simulink model "lotka_volterra"  (R2023a)
settings: Solver=VariableStepAuto  StartTime=0.0  StopTime=100  RelTol=1e-3
settings Model: Creator=vanes  LastModifiedBy=vanes
settings DataIOCC: ReturnWorkspaceOutputs=off  TimeSaveName=t

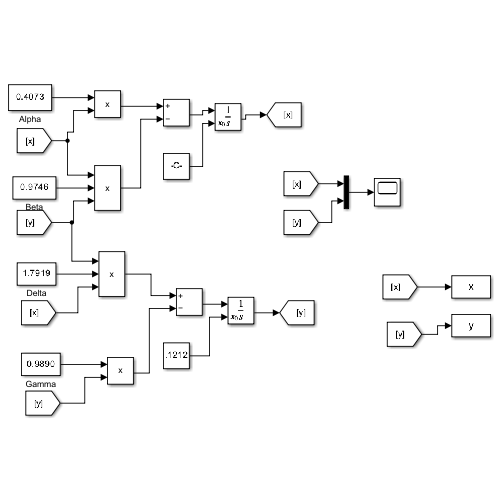
[thumbnail: Simulink's stored preview of the top-level diagram]
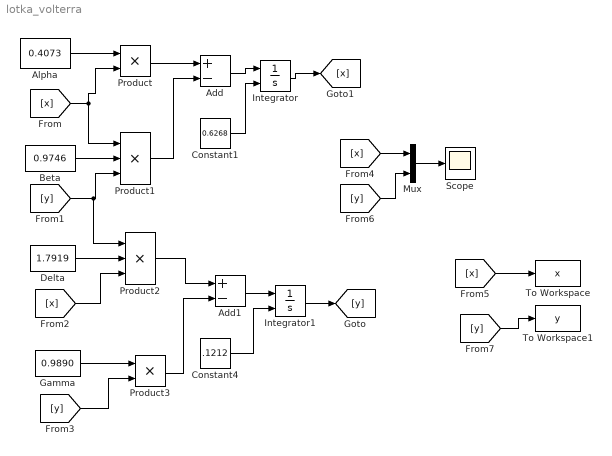
== system lotka_volterra ==
  Add : Sum  Inputs=+-
  Add1 : Sum  Inputs=+-
  Alpha : Constant  Value=0.4073
  Beta : Constant  Value=0.9746
  Constant1 : Constant  Value=0.6268
  Constant4 : Constant  Value=.1212
  Delta : Constant  Value=1.7919
  Gamma : Constant  Value=0.9890
  Integrator : Integrator  InitialConditionSource=external
  Integrator1 : Integrator  InitialConditionSource=external
  Mux : Mux  Inputs=2
  Product : Product
  Product1 : Product  Inputs=3
  Product2 : Product  Inputs=3
  Product3 : Product
  Scope : Scope
  To Workspace : ToWorkspace  VariableName=x  SampleTime=-1
  To Workspace1 : ToWorkspace  VariableName=y  SampleTime=-1
  wires:
  Alpha/1 -> Product/1
  [x] -> Product/2, Product1/1
  Beta/1 -> Product1/2
  [y] -> Product2/1, Product1/3
  Delta/1 -> Product2/2
  Product/1 -> Add/1
  Product1/1 -> Add/2
  Add/1 -> Integrator/1
  Integrator/1 -> [x]
  [x] -> Product2/3
  Gamma/1 -> Product3/1
  [y] -> Product3/2
  Constant4/1 -> Integrator1/2
  Integrator1/1 -> [y]
  Mux/1 -> Scope/1
  [x] -> Mux/1
  [x] -> To Workspace/1
  [y] -> Mux/2
  [y] -> To Workspace1/1
  Product2/1 -> Add1/1
  Product3/1 -> Add1/2
  Add1/1 -> Integrator1/1
  Constant1/1 -> Integrator/2
